simulink model "LookupTable1D_flat"  (R2017b)
settings: Solver=FixedStepDiscrete  StartTime=0.0  StopTime=10.0  FixedStep=0.200000  RelTol=1e-3  EnableMultiTasking=on
model workspace (MAT data in the model file):
  input_struct.time = [0; 0.2; 0.4; 0.6; 0.8; 1; 1.2; 1.4; 1.6; 1.8; 2; 2.2; 2.4; 2.6; 2.8; 3; 3.2; 3.4; 3.6; 3.8; 4; 4.2; 4.4; 4.6; 4.8; 5; 5.2; 5.4; 5.6; 5.8; 6; 6.2; 6.4; 6.6; 6.8; 7; 7.2; 7.4; 7.6; 7.8; 8; 8.2; 8.4; 8.6; 8.8; 9; 9.2; 9.4; 9.6; 9.8; 10; 10.2; 10.4; 10.6; 10.8; 11; 11.2; 11.4; 11.6; 11.8; 12; 12.2; 12.4; 12.6; 12.8; 13; 13.2; 13.4; 13.6; 13.8; 14; 14.2; 14.4; 14.6; 14.8; 15; 15.2; 15.4; 15.6; 15.8; 16; 16.2; 16.4; 16.6; 16.8; 17; 17.2; 17.4; 17.6; 17.8; 18; 18.2; 18.4; 18.6; 18.8; 19; 19.2; 19.4; 19.6; 19.8]
  input_struct.signals.name = 'In4'
  input_struct.signals.values = [28.8636260387; -24.2781234679; 62.3160916565; 6.56511775989; -29.8545792846; 87.8003124; 75.1885622986; 10.0312685797; 24.4950172002; 17.4089409063; -58.4515414534; -39.7507339441; -5.81533029648; -53.9023679577; 68.8617585391; -61.0471420866; -54.8156438055; -65.8583905704; -54.4671404367; -12.8602631792; -37.7795426699; 84.6759284206; -13.9585217341; -63.0367359752; 80.976193736; 95.9496756712; -12.2260053748; -77.7761553119; -48.3870608176; -18.2560307775; 18.9792148017; -47.5576504438; 20.5686178764; 42.2431560867; -55.6506531966; -76.5164698288; -40.6648253563; -36.2443396148; -15.1666480572; 1.57165693222; -82.896840582; -47.5035530603; 60.2029245539; -94.1559444876; 85.7708278956; 46.0661725711; -2.27820523928; 15.7050122047; -52.5432840457; -8.23023436401; 92.6177078574; 9.36114374779; 4.2271661608; -53.6811226583; -2.22045121597; 24.8120176347; 35.8271081731; -20.8969568663; -26.5126702911; 97.5964006323; -92.4522267521; 77.0336016405; 82.6573655278; 59.236774717; -80.2575442689; -47.6257632259; -32.9286320074; 35.9455902755; -72.6893725289; 44.2454997163; -78.6476276786; 30.7514697337; -1.16521267215; 55.8103446463; 43.0074156801; 80.7441121113; 78.1845008662; -33.1673894525; 39.749166467; -60.4380346628; -93.8918107391; 48.8148520735; 0.00448711804017; -4.01557177079; 80.9444476135; 21.9733296845; 23.5332779177; 71.8884611292; 61.0978849059; 15.3443031229; -63.415506117; -52.0135978863; 77.3023866152; -94.2651695072; -2.01972229756; -66.4145708635; 95.7361299282; 42.5388943358; 0.0943248309686; -5.78232509161]
  input_struct.signals.dimensions = 1
settings Model: Creator=hbourbou  LastModifiedBy=hbourbou
settings DataIOCC: LimitDataPoints=on  SaveFormat=StructureWithTime
settings OptimizationCC: LifeSpan=inf
settings DebuggingCC: SFUnexpectedBacktrackingDiag=warning  SFNoUnconditionalDefaultTransitionDiag=warning  SFExecutionAtInitializationDiag=none
settings HardwareCC: ProdBitPerSizeT=32  ProdBitPerPtrDiffT=32  ProdWordSize=32  ProdHWDeviceType=Specified
settings ModelReferenceCC: PropagateSignalLabelsOutOfModel=off
settings CodeAppCC: StateflowObjectComments=on
settings GRTTargetCC: TargetLangStandard=C89/C90 (ANSI)
settings ConfigComp: CovMetricSettings=dw  CovHtmlReporting=on  CovSaveCumulativeToWorkspaceVar=on  CovSaveSingleToWorkspaceVar=on  CovExternalEMLEnable=off

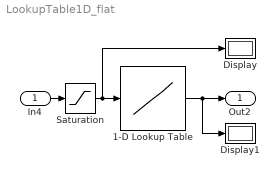
== system LookupTable1D_flat ==
  In4 : Inport
  1-D Lookup Table : Lookup_n-D  NumberOfTableDimensions=1  BreakpointsForDimension1=[0:0.1:2*pi]  Table=cos([0:0.1:2*pi])  InterpMethod=Flat  ExtrapMethod=Clip  InternalRulePriority=Speed  RndMeth=Simplest  InputSameDT=on
  Display : Display
  Display1 : Display
  Saturation : Saturate  UpperLimit=1.5  LowerLimit=-1.5
  Out2 : Outport
  wires:
  1-D Lookup Table/1 -> Display1/1, Out2/1
  In4/1 -> Saturation/1
  Saturation/1 -> Display/1, 1-D Lookup Table/1
